simulink model "NNEntradaRadom"  (Simulink 7.3)
settings: Solver=ode45  StartTime=0.0  StopTime=100  RelTol=1e-3
undefined symbols (not defined in the file or in its folder): now
libraries: simulink_extras x3, neural x1
settings Model: Creator=marco  LastModifiedBy=Iuri
settings DebuggingCC: SaveWithParameterizedLinksMsg=none

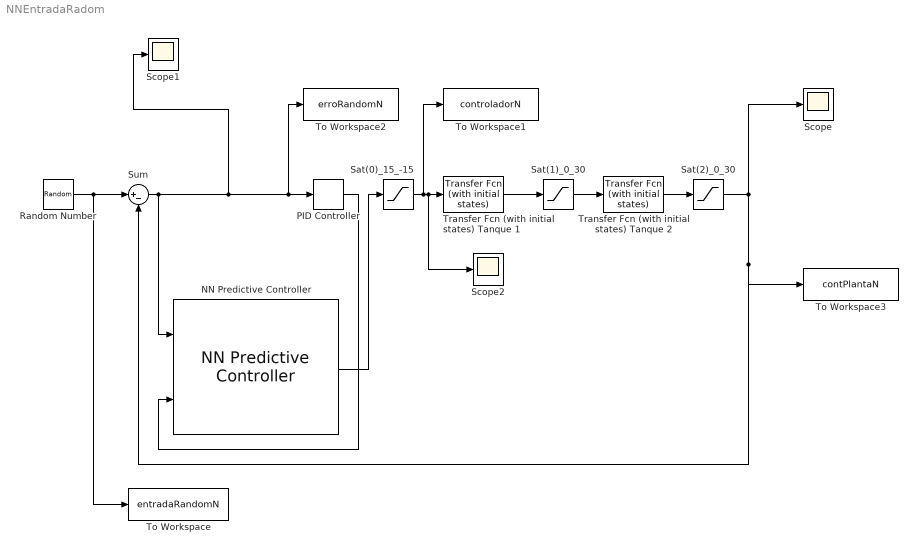
== system NNEntradaRadom ==
  NN Predictive Controller : neural/Control Systems/NN Predictive Controller  SystemSampleTime=-1  csrchfun=csrchbac  trainfun=trainlm
  PID Controller : simulink_extras/Additional Linear/PID Controller  SystemSampleTime=-1  P=10.7  I=0.5  D=0
  Random Number : RandomNumber  Mean=15  Variance=15  Seed=round(now)  SampleTime=500
  Sat(0)_15_-15 : Saturate  UpperLimit=15  LowerLimit=-15  SampleTime=0.1
  Sat(1)_0_30 : Saturate  UpperLimit=30  LowerLimit=0  SampleTime=0.1
  Sat(2)_0_30 : Saturate  UpperLimit=30  LowerLimit=0  SampleTime=0.1
  Scope : Scope
  Scope1 : Scope
  Scope2 : Scope
      settings: SaveName=ScopeData2
  Sum : Sum  Inputs=|+-  OutDataType=fixdt(1, 16)  OutScaling=2^0  SampleTime=0.1
  To Workspace : ToWorkspace  VariableName=entradaRandomN  SampleTime=0.1  SaveFormat=Array
  To Workspace1 : ToWorkspace  VariableName=controladorN  SampleTime=0.1  SaveFormat=Array
  To Workspace2 : ToWorkspace  VariableName=erroRandomN  SampleTime=0.1  SaveFormat=Array
  To Workspace3 : ToWorkspace  VariableName=contPlantaN  SampleTime=0.1  SaveFormat=Array
  Transfer Fcn (with initial states) Tanque 1 : simulink_extras/Additional Linear/Transfer Fcn (with initial states)  SystemSampleTime=-1  N=[0.2964]  D="[1  0.0656]"  X0=0
  Transfer Fcn (with initial states) Tanque 2 : simulink_extras/Additional Linear/Transfer Fcn (with initial states)  SystemSampleTime=-1  N=[0.0656]  D="[1  0.0656]"  X0=0
  wires:
  Transfer Fcn (with initial states) Tanque 1/1 -> Sat(1)_0_30/1
  PID Controller/1 -> NN Predictive Controller/2
  Sum/1 -> To Workspace2/1, PID Controller/1, Scope1/1, NN Predictive Controller/1
  Transfer Fcn (with initial states) Tanque 2/1 -> Sat(2)_0_30/1
  Sat(0)_15_-15/1 -> To Workspace1/1, Transfer Fcn (with initial states) Tanque 1/1, Scope2/1
  Random Number/1 -> Sum/1, To Workspace/1
  Sat(1)_0_30/1 -> Transfer Fcn (with initial states) Tanque 2/1
  Sat(2)_0_30/1 -> Sum/2, To Workspace3/1, Scope/1
  NN Predictive Controller/1 -> Sat(0)_15_-15/1
